simulink model "OneToOne"  (R2014a)
settings: Solver=ode45  StartTime=0.0  StopTime=10.0  RelTol=1e-3
values from neighbouring files (symbols this model uses):
  I = 1/12*m*((2*ry1)^2 + (2*rx1)^2)    (= 7.53502955357)    [parameters1.m]
  inputBound = [minInput maxInput]    [parameters1.m]
  K = [1000 1000 1000 10 10 1 1]    [parameters1.m]
  k1m = 50    [parameters1.m]
  k1x = 100    [parameters1.m]
  k1y = 100    [parameters1.m]
  k2m = 25    [parameters1.m]
  k2x = 60    [parameters1.m]
  k2y = 60    [parameters1.m]
  m = 46.27    [parameters1.m]
  rx1 = rx01    [Minimizer.m]    (also in parameters1.m = -0.635)
  rx2 = rx02    [Minimizer.m]    (also in parameters1.m = -0.635)
  ry1 = ry01    [Minimizer.m]    (also in parameters1.m = 0.2921)
  ry2 = ry02    [Minimizer.m]    (also in parameters1.m = -0.2921)
settings Model: Creator=propagator  LastModifiedBy=propagator
settings OptimizationCC: SimCompilerOptimization=On
settings HardwareCC: ProdBitPerLong=64  ProdBitPerPointer=64  ProdIntDivRoundTo=Zero  ProdEndianess=LittleEndian  ProdWordSize=64  ProdHWDeviceType=Intel->x86-64
settings ModelReferenceCC: EnableParallelModelReferenceBuilds=on
settings RTWCC: BuildConfiguration=Faster Runs  TargetLang=C++
settings GRTTargetCC: MultiInstanceERTCode=on  CodeInterfacePackaging=C++ class

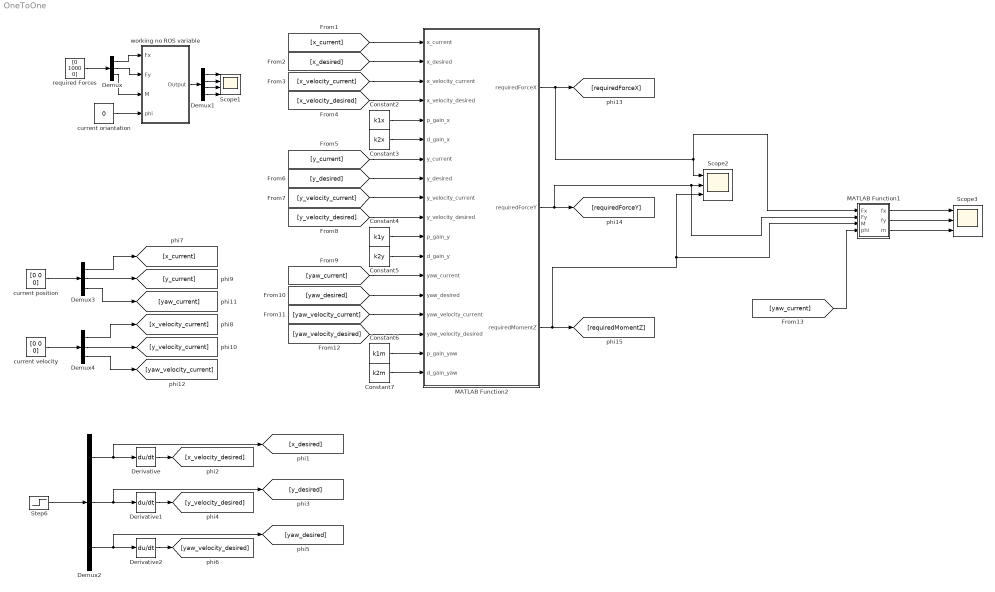
== system OneToOne ==
  Constant2 : Constant  Value=k1x
  Constant3 : Constant  Value=k2x
  Constant4 : Constant  Value=k1y
  Constant5 : Constant  Value=k2y
  Constant6 : Constant  Value=k1m
  Constant7 : Constant  Value=k2m
  Demux{,2..4} (4 alike) : Demux  Outputs=3
  Demux1 : Demux
  Derivative : Derivative
  Derivative1 : Derivative
  Derivative2 : Derivative
  MATLAB Function1 : MATLAB Function  TreatAsAtomicUnit=on
  MATLAB Function2 : MATLAB Function  TreatAsAtomicUnit=on
  Scope1 : Scope  NumInputPorts=4
      settings: YMin=-69.9983~-23.65~69.9983~39.25  YMax=-69.9983~-23.65~69.9983~39.25
  Scope2 : Scope  NumInputPorts=3
      settings: YMin=-3~905~-185  YMax=0~940~-155
  Scope3 : Scope  NumInputPorts=3
      settings: YMin=-3~905~-185  YMax=0~940~-155  SaveName=ScopeData2
  Step6 : Step  Before=[0;0;0]  After=[0;10;0]  SampleTime=0
  current oriantation : Constant  Value=0
  current position : Constant  Value=[0 0 0]
  current velocity : Constant  Value=[0 0 0]
  required Forces : Constant  Value=[0 1000 0]
  working no ROS variable : Subsystem  mask{rx1=rx1, rx2=rx2, ry1=ry1, ry2=ry2, C=K, inputBound=inputBound, m=m, I=I}
      mask prompts: C "Performance Gain"; inputBound "Input Bounds"; m "Boat Mass"; I "Boat Inertia"
      mask TypeOptions m: Constant6/Value
      mask TypeOptions I: Constant7/Value
  wires:
  Demux/3 -> working no ROS variable/3(M)
  Demux/2 -> working no ROS variable/2(Fy)
  Demux/1 -> working no ROS variable/1(Fx)
  required Forces/1 -> Demux/1
  current oriantation/1 -> working no ROS variable/4(phi)
  Demux1/4 -> Scope1/4
  Demux1/3 -> Scope1/3
  Demux1/2 -> Scope1/2
  Demux1/1 -> Scope1/1
  working no ROS variable/1(Output) -> Demux1/1
  Constant3/1 -> MATLAB Function2/6(d_gain_x)
  Constant2/1 -> MATLAB Function2/5(p_gain_x)
  Constant6/1 -> MATLAB Function2/17(p_gain_yaw)
  Constant7/1 -> MATLAB Function2/18(d_gain_yaw)
  Constant5/1 -> MATLAB Function2/12(d_gain_y)
  Constant4/1 -> MATLAB Function2/11(p_gain_y)
  [x_current] -> MATLAB Function2/1(x_current)
  [x_desired] -> MATLAB Function2/2(x_desired)
  [x_velocity_current] -> MATLAB Function2/3(x_velocity_current)
  [x_velocity_desired] -> MATLAB Function2/4(x_velocity_desired)
  [yaw_velocity_desired] -> MATLAB Function2/16(yaw_velocity_desired)
  [yaw_velocity_current] -> MATLAB Function2/15(yaw_velocity_current)
  [yaw_desired] -> MATLAB Function2/14(yaw_desired)
  [yaw_current] -> MATLAB Function2/13(yaw_current)
  [y_velocity_desired] -> MATLAB Function2/10(y_velocity_desired)
  [y_velocity_current] -> MATLAB Function2/9(y_velocity_current)
  [y_desired] -> MATLAB Function2/8(y_desired)
  [y_current] -> MATLAB Function2/7(y_current)
  MATLAB Function2/2(requiredForceY) -> MATLAB Function1/2(Fy), Scope2/2, [requiredForceY]
  MATLAB Function2/3(requiredMomentZ) -> MATLAB Function1/3(M), Scope2/3, [requiredMomentZ]
  MATLAB Function2/1(requiredForceX) -> MATLAB Function1/1(Fx), Scope2/1, [requiredForceX]
  Demux2/3 -> [yaw_desired], Derivative2/1
  Demux2/2 -> [y_desired], Derivative1/1
  Derivative2/1 -> [yaw_velocity_desired]
  Derivative1/1 -> [y_velocity_desired]
  Demux2/1 -> [x_desired], Derivative/1
  Step6/1 -> Demux2/1
  Derivative/1 -> [x_velocity_desired]
  Demux3/1 -> [x_current]
  Demux3/2 -> [y_current]
  Demux3/3 -> [yaw_current]
  Demux4/1 -> [x_velocity_current]
  Demux4/2 -> [y_velocity_current]
  Demux4/3 -> [yaw_velocity_current]
  current velocity/1 -> Demux4/1
  current position/1 -> Demux3/1
  MATLAB Function1/1(fx) -> Scope3/1
  MATLAB Function1/2(fy) -> Scope3/2
  MATLAB Function1/3(m) -> Scope3/3
  [yaw_current] -> MATLAB Function1/4(phi)

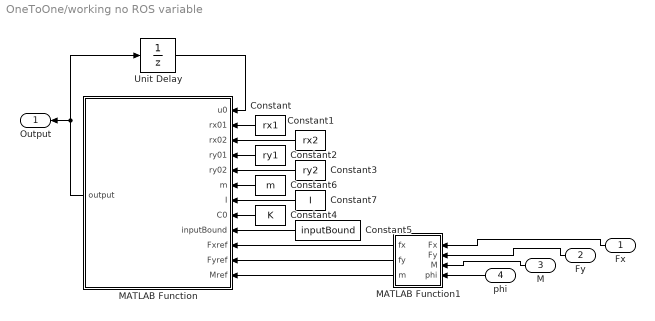
== system OneToOne/working no ROS variable ==
  Fx : Inport
  Fy : Inport  Port=2
  M : Inport  Port=3
  phi : Inport  Port=4
  Constant : Constant  Value=rx1
  Constant1 : Constant  Value=rx2
  Constant2 : Constant  Value=ry1
  Constant3 : Constant  Value=ry2
  Constant4 : Constant  Value=K
  Constant5 : Constant  Value=inputBound
  Constant6 : Constant  Value=m
  Constant7 : Constant  Value=I
  MATLAB Function : MATLAB Function  TreatAsAtomicUnit=on
  MATLAB Function1 : MATLAB Function  TreatAsAtomicUnit=on
  Unit Delay : UnitDelay  InitialCondition=[0;0;0;0]  SampleTime=-1
  Output : Outport
  wires:
  Constant/1 -> MATLAB Function/2(rx01)
  Constant1/1 -> MATLAB Function/3(rx02)
  Constant2/1 -> MATLAB Function/4(ry01)
  Constant4/1 -> MATLAB Function/8(C0)
  Unit Delay/1 -> MATLAB Function/1(u0)
  MATLAB Function/1(output) -> Unit Delay/1, Output/1
  Constant5/1 -> MATLAB Function/9(inputBound)
  Constant3/1 -> MATLAB Function/5(ry02)
  MATLAB Function1/3(m) -> MATLAB Function/12(Mref)
  MATLAB Function1/2(fy) -> MATLAB Function/11(Fyref)
  MATLAB Function1/1(fx) -> MATLAB Function/10(Fxref)
  Fy/1 -> MATLAB Function1/2(Fy)
  Fx/1 -> MATLAB Function1/1(Fx)
  M/1 -> MATLAB Function1/3(M)
  phi/1 -> MATLAB Function1/4(phi)
  Constant6/1 -> MATLAB Function/6(m)
  Constant7/1 -> MATLAB Function/7(I)

== matlab function OneToOne/MATLAB Function2 ==
  data: x_current input; requiredForceX output; x_desired input; x_velocity_current input; x_velocity_desired input; p_gain_x input; d_gain_x input; y_current input; y_desired input; y_velocity_current input; y_velocity_desired input; p_gain_y input; d_gain_y input; yaw_current input; yaw_desired input; yaw_velocity_current input; yaw_velocity_desired input; p_gain_yaw input; d_gain_yaw input; requiredForceY output; requiredMomentZ output
function [requiredForceX,requiredForceY,requiredMomentZ] = fcn(x_current,x_desired,x_velocity_current,x_velocity_desired, p_gain_x,d_gain_x,...
                            y_current,y_desired,y_velocity_current,y_velocity_desired, p_gain_y, d_gain_y,...
                            yaw_current,yaw_desired,yaw_velocity_current,yaw_velocity_desired, p_gain_yaw, d_gain_yaw)

requiredForceX = p_gain_x * (x_desired - x_current) + d_gain_x * (x_velocity_desired - x_velocity_current);
requiredForceY = p_gain_y * (y_desired - y_current) + d_gain_y * (y_velocity_desired - y_velocity_current);
requiredMomentZ = p_gain_yaw * (yaw_desired - yaw_current) + d_gain_yaw * (yaw_velocity_desired - yaw_velocity_current);
end

== matlab function OneToOne/MATLAB Function1 ==
  data: Fx input; fx output; Fy input; M input; fy output; m output; phi input
function [fx,fy,m] = fcn(Fx,Fy,M, phi)
%#codegen

R = [cosd(phi) -sind(phi) 0;...
        sind(phi)  cosd(phi) 0;...
        0           0       1];
    
    FxyM = R'*[Fx;Fy;M];
    
    fx = FxyM(1);
    fy = FxyM(2);
    m = FxyM(3);
    
end

== matlab function OneToOne/working no ROS variable/MATLAB Function ==
  data: u0 input; output output; rx01 input; rx02 input; ry01 input; ry02 input; m input; I input; C0 input; inputBound input; Fxref input; Fyref input; Mref input
function output = Minimizer(u0, rx01, rx02, ry01, ry02, m, I, C0, inputBound, Fxref, Fyref, Mref)

rx1 = rx01; rx2 = rx02;
ry1 = ry01; ry2 = ry02;

C = C0;

%Fxref = Fx; Fyref = Fy; Mref  = M;

gridNum = 10;

grid = boundGrid(inputBound, gridNum, rx1,ry1);

u1 = getMinFromGrid(grid, u0, Fxref, Fyref, Mref, rx1, rx2, ry1, ry2, C, m, I);

% u1 = u0;

% %     for k = 1:20
% %         h = getDirection(u1, u0, Fxref, Fyref, Mref, rx1, rx2, ry1, ry2, C);
% %         alpha = getStepSize(u1, u0, h, Fxref, Fyref, Mref, rx1, rx2, ry1, ry2, C);
% %         u1 = u1 + alpha*h;
% %         u1 = checkInputBound(u1,inputBound);
% %     end
    
    output = u1;

end

function output = getMinFromGrid(grid, preinput, Fxref, Fyref, Mref, rx1, rx2, ry1, ry2, C, m, I)

[ii, iii] = size(grid);
v0 = costFunction(grid(1,:), preinput, Fxref, Fyref, Mref, rx1, rx2, ry1, ry2, C, m, I);

output = [grid(1,1);grid(1,2);grid(1,3);grid(1,4)];

for i = 1:ii
    for j = 1:ii
        for k = 1:ii
            for l = 1:ii
                input = [grid(i,1);grid(j,2);grid(k,3);grid(l,4)];
                v1 = costFunction(input,preinput, Fxref, Fyref, Mref, rx1, rx2, ry1, ry2, C, m, I);
                if v0 > v1
                    v0 = v1;
                    output = input;
                else
                end
            end
        end
    end
end

end

function output = checkInputBound(input,inputBound)
k = [0;0;0;0];
    for i = 1:length(input)
        k(i) = sat(input(i),inputBound(i,:));
    end
    output = k;
end

function output = boundGrid(inputBound, gridNum, rx1,ry1)

p = gridNum;

current_port_servo_angle =    [0.2664;0.1837;0.1010;0.0184;-0.0643;-0.1470;-0.2296;-0.3123;-0.3950;-0.4777;...
-0.5603;-0.6430;-0.7257;-0.8084;-0.8910;-0.9737;-1.0564;-1.1054;-1.1391;-1.2217]*180/pi;                      %linspace(inputBound(1,1),inputBound(1,2),p)';
current_port_thruster_force =        [39.25;30;20;10;5;0;-5;-10;-15;-23.65;zeros(10,1)];                                                             %linspace(inputBound(2,1),inputBound(2,2),p)';
current_starboard_servo_angle =    [0.2664;0.1837;0.1010;0.0184;-0.0643;-0.1470;-0.2296;-0.3123;-0.3950;-0.4777;...
-0.5603;-0.6430;-0.7257;-0.8084;-0.8910;-0.9737;-1.0564;-1.1054;-1.1391;-1.2217]*-180/pi;                      %linspace(inputBound(3,1),inputBound(3,2),p)';
current_starboard_thruster_force =        [39.25;30;20;10;5;0;-5;-10;-15;-23.65;zeros(10,1)];                                                            %linspace(inputBound(4,1),inputBound(4,2),p)';

%i = atan(rx1/ry1)*180/pi;

output = [current_port_servo_angle, current_port_thruster_force, current_starboard_servo_angle, current_starboard_thruster_force];%;...
%           inputBound(1,1),  0,      inputBound(3,1),  0;...
%              0,    100,    0,    100;...%];
%              0,   -100,    0,   -100]; %...
%             i,    0,    i,    0];

% p = gridNum;
% 
% theta1 =    linspace(inputBound(1,1),inputBound(1,2),p)';
% f1 =        linspace(inputBound(2,1),inputBound(2,2),p)';
% theta2 =    linspace(inputBound(3,1),inputBound(3,2),p)';
% f2 =        linspace(inputBound(4,1),inputBound(4,2),p)';
% 
% %i = atan(rx1/ry1)*180/pi;
% 
% output = [theta1, f1, theta2, f2;...
%           inputBound(1,1),  0,      inputBound(3,1),  0;...
%              0,    100,    0,    100;...%];
%              0,   -100,    0,   -100]; %...
% %             i,    0,    i,    0];

end

function output = sat(input, bound)

    if input < bound(1)
        output = bound(1);
    elseif input > bound(2)
        output = bound(2);
    else
        output = input;
    end

end

function output = getStepSize(input, preinput, h, Fxref, Fyref, Mref, rx1, rx2, ry1, ry2, C, m, I)

    alpha = .001;
    
    u0 = input;
    u1 = input + alpha*h;
    
    v0 = costFunction( u0, preinput, Fxref, Fyref, Mref, rx1, rx2, ry1, ry2, C, m, I );
    v1 = costFunction( u1, preinput, Fxref, Fyref, Mref, rx1, rx2, ry1, ry2, C, m, I);

    while v1 <= v0 && v1 ~= 0
        alpha = alpha + .001;
        u1 = input + alpha*h;
        v0 = v1;
        v1 = costFunction( u1, preinput, Fxref, Fyref, Mref, rx1, rx2, ry1, ry2, C, m, I );
    end
    
    v0 = v1;
    alpha = .0015;

    while v1 <= v0  && v1 ~= 0
        alpha = alpha - 0.0001;
        u1 = input + alpha*h;
        v0 = v1;
        v1 = costFunction( u1, preinput, Fxref, Fyref, Mref, rx1, rx2, ry1, ry2, C, m, I );
    end


    output = alpha;

end

function output = costFunction(input, preinput, Fxref, Fyref, Mref, rx1, rx2, ry1, ry2, C, m, I)

    theta1  = input(1);
    f1      = input(2);
    theta2  = input(3);
    f2      = input(4);
    
    pretheta1   = preinput(1);
    pretheta2   = preinput(3);

    Fx = f1*cosd(theta1) + f2*cosd(theta2);
    Fy = f1*sind(theta1) + f2*sind(theta2);
    M = -rx1*f1*sind(theta1) + ry1*f1*cosd(theta1) - rx2*f2*sind(theta2)...
        + ry2*f2*cosd(theta2);

    output = C(1)*(Fx-Fxref)^2 +...
        C(2)*(Fy-Fyref)^2 +...
        C(3)*(M-Mref)^2  +...
        C(4)*f1^2 +...
        C(5)*f2^2 +...
        C(6)*(theta1 - pretheta1)^2 +...
        C(7)*(theta2 - pretheta2)^2;% +...
%         C(5)*theta1^2 +...
%         C(5)*theta2^2;

end

function output = getDirection(input, preinput, Fxref, Fyref, Mref, rx1, rx2, ry1, ry2, C, m, I)

hsd = SteepestDescent(input, preinput, Fxref, Fyref, Mref, rx1, rx2, ry1, ry2, C, m, I);

output = zeros(4,1);

    for i = 1:length(hsd)
        output(i) = hsd(i);
    end
    
end

function output = SteepestDescent(input, preinput, Fxref, Fyref, Mref, rx1, rx2, ry1, ry2, C, m, I)

theta1  = input(1);
f1      = input(2);
theta2  = input(3);
f2      = input(4);

pretheta1   = preinput(1);
pretheta2   = preinput(3);

dVdtheta1 = C(3)*(f1*ry1*cosd(theta1)...
    - f1*rx1*sind(theta1))*(f1*rx1*cosd(theta1)...
    - Mref + f2*rx2*cosd(theta2) + f1*ry1*sin(theta1)...
    + f2*ry2*sind(theta2)) - C(6)*(pretheta1 - theta1)...
    - C(2)*f1*sind(theta1)*(f1*cosd(theta1) - Fyref + f2*cosd(theta2))...
    + C(1)*f1*cosd(theta1)*(Fxref + f1*sind(theta1) + f2*sind(theta2));

dVdf1 = C(4)*f1 + C(1)*sind(theta1)*(Fxref + f1*sin(theta1)...
    + f2*sind(theta2)) + C(2)*cosd(theta1)*(f1*cosd(theta1) - Fyref...
    + f2*cosd(theta2)) + C(3)*(rx1*cosd(theta1)...
    + ry1*sind(theta1))*(f1*rx1*cosd(theta1) - Mref + f2*rx2*cosd(theta2)...
    + f1*ry1*sind(theta1) + f2*ry2*sind(theta2));

dVdtheta2 = C(3)*(f2*ry2*cosd(theta2)...
    - f2*rx2*sind(theta2))*(f1*rx1*cosd(theta1)...
    - Mref + f2*rx2*cosd(theta2) + f1*ry1*sind(theta1)...
    + f2*ry2*sind(theta2)) - C(7)*(pretheta2 - theta2)...
    - C(2)*f2*sind(theta2)*(f1*cosd(theta1) - Fyref + f2*cosd(theta2))...
    + C(1)*f2*cosd(theta2)*(Fxref + f1*sind(theta1) + f2*sind(theta2));

dVdf2 = C(5)*f2 + C(1)*sind(theta2)*(Fxref + f1*sind(theta1)...
    + f2*sind(theta2)) + C(2)*cosd(theta2)*(f1*cosd(theta1) - Fyref...
    + f2*cosd(theta2)) + C(3)*(rx2*cosd(theta2)...
    + ry2*sind(theta2))*(f1*rx1*cosd(theta1) - Mref + f2*rx2*cosd(theta2)...
    + f1*ry1*sind(theta1) + f2*ry2*sind(theta2));
 
output = -[dVdtheta1; dVdf1; dVdtheta2; dVdf2];

end

== matlab function OneToOne/working no ROS variable/MATLAB Function1 ==
  data: Fx input; fx output; Fy input; M input; fy output; m output; phi input
function [fx,fy,m] = fcn(Fx,Fy,M, phi)
%#codegen

R = [cosd(phi) -sind(phi) 0;...
        sind(phi)  cosd(phi) 0;...
        0           0       1];
    
    FxyM = R'*[Fx;Fy;M];
    
    fx = FxyM(1);
    fy = FxyM(2);
    m = FxyM(3);
    
end
